simulink model "vibrating_sys"  (Simulink 8.3)
settings: Solver=ode4  SolverMode=SingleTasking  StartTime=0.0  StopTime=20  FixedStep=1e-2  MaxStep=1e-2  RelTol=1e-2
values from neighbouring files (symbols this model uses):
  D = D+diag([0.4,0.5*ones(1,209),0.4])    [ModeloVI.m]    (also in Modelo_I.m = [4,1;1,5]; Modelo_II.m = [-2.0374,9.0183,6.6374;0.3073,4.4470,-7.3132;      3.1506 ,-; Modelo_III.m = [7.66,2.45,2.1;0.23,1.04,0.223;0.60,0.756,0.658]; Modelo_IV.m = D+diag([1.3525,1.3274,0.9456,1.1536]))
  F1 = Ftild    [Modelo_III.m]
  F2 = D_EVA_disco(A,B,r,q)    [Modelo_III.m]
  K = K+200*diag([0.5,ones(1,209),0.5])    [ModeloVI.m]    (also in Modelo_I.m = [8,ese;-ese,9]; Modelo_II.m = [-8.3151,-3.9655,-8.0925;-6.7220,-9.7664,-7.0697;     -3.515; Modelo_III.m = [121,18.9,15.9;0,2.7,0.145;11.9,3.64,15.5]; Modelo_IV.m = K+diag([1.7824,1.0287,2.8360,1.9130]))
  M = eye(211)    [ModeloVI.m]    (also in Modelo_I.m = [10,0;0,11]; Modelo_II.m = [-7.6593,-5.0754,0.9311;6.2936,3.1457,1.2384;     -3.5029,-2; Modelo_III.m = [17.6,1.28,2.89; 1.28,0.824,0.413;2.89,0.413,0.725]; Modelo_IV.m = M+diag([1.4685,2.6938,2.7061,2.1876]))
  N = eye(211,1)    [ModeloVI.m]    (also in Modelo_I.m = [1;-1]; Modelo_II.m = eye(3); Modelo_III.m = [1;1;1]; Modelo_IV.m = [1;2;1;-1])
settings Model: Creator=Jose  LastModifiedBy=Dell  CovSFcnEnable=on
settings OptimizationCC: BlockReduction=off  BooleanDataType=off  ExpressionDepthLimit=2147483647
settings DebuggingCC: SaveWithParameterizedLinksMsg=none  SignalResolutionControl=TryResolveAllWithWarning  SolverPrmCheckMsg=none  MultiTaskDSMMsg=warning  MultiTaskCondExecSysMsg=none  FrameProcessingCompatibilityMsg=error
settings HardwareCC: TargetLongLongMode=on  TargetIntDivRoundTo=Zero  TargetEndianess=LittleEndian  TargetHWDeviceType=MATLAB Host  ProdEqTarget=off
settings GRTTargetCC: CombineOutputUpdateFcns=on  GRTInterface=off

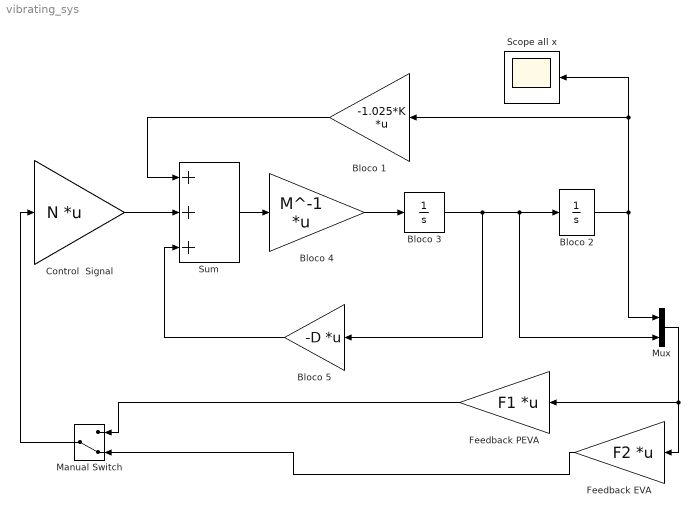
== system vibrating_sys ==
  Bloco 1 : Gain  Gain=-1.025*K  Multiplication=Matrix(K*u)
  Bloco 2 : Integrator  InitialCondition=[1;0;0]
  Bloco 3 : Integrator
  Bloco 4 : Gain  Gain=M^-1  Multiplication=Matrix(K*u)
  Bloco 5 : Gain  Gain=-D  Multiplication=Matrix(K*u)
  Control  Signal : Gain  Gain=N  Multiplication=Matrix(K*u)
  Feedback EVA : Gain  Gain=F2  Multiplication=Matrix(K*u)
  Feedback PEVA : Gain  Gain=F1  Multiplication=Matrix(K*u)
  Manual Switch : ManualSwitch  CurrentSetting=0
  Mux : Mux  Inputs=2
  Scope all x : Scope
      settings: TimeRange=15  YMin=-15  YMax=15  SaveName=ht_EVA
  Sum : Sum  Inputs=+++
  wires:
  Bloco 1/1 -> Sum/1
  Sum/1 -> Bloco 4/1
  Bloco 4/1 -> Bloco 3/1
  Bloco 2/1 -> Mux/1, Scope all x/1, Bloco 1/1
  Bloco 3/1 -> Bloco 5/1, Mux/2, Bloco 2/1
  Bloco 5/1 -> Sum/3
  Mux/1 -> Feedback EVA/1, Feedback PEVA/1
  Control  Signal/1 -> Sum/2
  Feedback PEVA/1 -> Manual Switch/1
  Manual Switch/1 -> Control  Signal/1
  Feedback EVA/1 -> Manual Switch/2
